simulink model "estimation_over_network"  (R2022b)
settings: Solver=VariableStepAuto  StartTime=0.0  StopTime=T  MaxStep=MaxStep  RelTol=RelTol
values from neighbouring files (symbols this model uses):
  J = 20    [initialization.m]
  T = 10    [initialization.m]
  X0 = [1;0.6;1]    [initialization.m]
libraries: HyEQ_Library x3
settings Model: Creator=tom  LastModifiedBy=tom

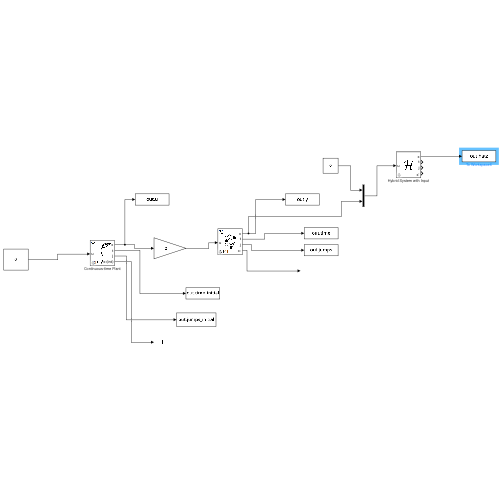
[thumbnail: Simulink's stored preview of the top-level diagram]
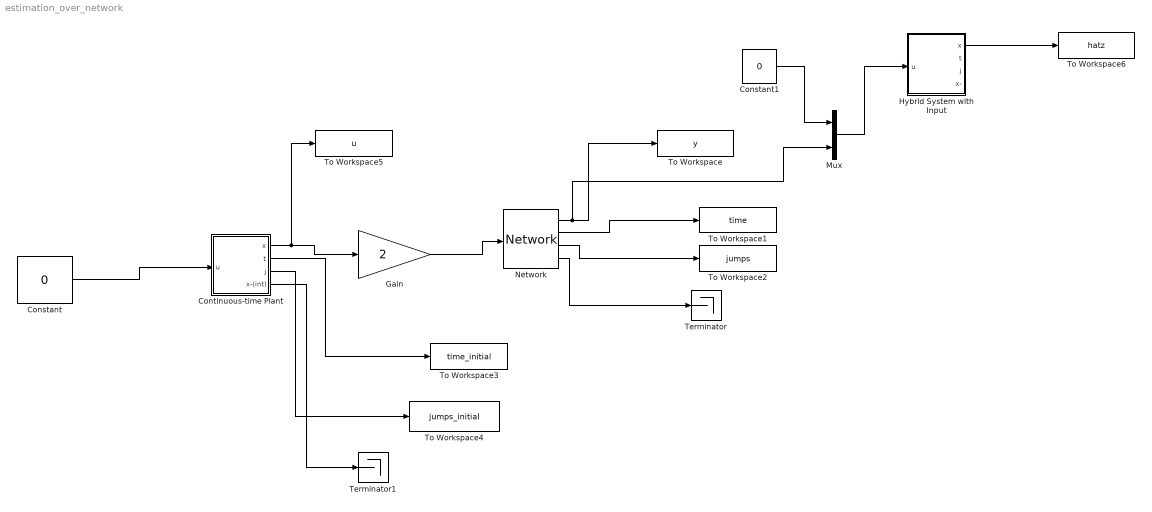
== system estimation_over_network ==
  Constant : Constant  Value=0
  Constant1 : Constant  Value=0
  Continuous-time Plant : Subsystem  LoadFcn=set_param(gcb,'LinkStatus','none')  mask(Continuous Process){z0=X0, input_dim=1, parameters=[], T=T}
      mask prompts: z0 "Initial State (column vector)"; input_dim "Input dimension (nonnegative integer)"; T "Flow Horizon (nonnegative real)"
      mask help:
      | To define the continuous process:
      | 1. Select the block,
      | 2. "Look inside" the block: Either open the context menu and select Mask > Look Under Mask, or click the arrow in the bottom-left corner of the block.
      | 3. Edit the "flow map f" block to define the continuous dynamics.
      | 4. Edit the "flow set C" block to define the region where the continuous process is allowed to flow.
      mask init:
      | state_dim = size(z0, 1);
      settings: CopyFcn=|
      | set_param(gcb,'LinkStatus','none'),
      | set_param(gcs, 'MaxStep', 'MaxStep', 'RelTol', 'RelTol','StopTime', 'T')
      mask Help: eval hybrid.internal.openHelp('Example_vehicle_on_path')
      mask TypeOptions T: Integrator System/T
      mask DialogControl Control2 Prompt: CPS Components Documentation
      mask DialogControl Control2 Callback: hybrid.internal.openHelp('CPS_Components')
      mask DialogControl ParameterGroupVar Prompt: Configuration
      mask Display:
      | image('Cplant.jpg')
      | port_label('output', 1, 'x')
      | port_label('output', 2, 't')
      | port_label('output', 3, 'j')
      | port_label('output', 4, 'x-(int)')
      | port_label('input', 1, 'u')
  Gain : Gain  Gain=2
  Hybrid System with Input : Subsystem  LoadFcn=set_param(gcb,'LinkStatus','none')  mask(Hybrid System with Inputs){x0=0, input_dim=6, parameters=[], T=T, J=J, rule=Jump}
      mask prompts: x0 "Initial Condition (column vector)"; input_dim "Input Dimension (positive integer)"; T "Flow Horizon (nonnegative real)"; J "Jump Horizon (nonnegative integer)"; rule "Flow/Jump Priorty Rule"
      mask help:
      | To modify (f, g, C, D) for this block, "Look inside" the block mask by either clicking the down arrow in the lower-left corner or selecting "Mask" > "Look Under Mask" from the context menu.
      |
      | For instructions how to use this block, see the
      mask init:
      | state_dim = numel(x0);
      settings: CopyFcn=|
      | set_param(gcb,'LinkStatus','none'),
      | set_param(gcs, 'MaxStep', 'MaxStep', 'RelTol', 'RelTol','StopTime', 'T')
      mask Help:
      | To modify (f, g, C, D) for this block, "Look inside" the block mask by either clicking the down arrow in the lower-left corner or selecting "Mask" > "Look Under Mask" from the context menu.
      | 
      | The value given in the 'parameters' field is passed as the last input argument for f, g, C, and D. Any MATLAB object can be used, but we recommend using a struct. For example, in the initialization script, a parameters struct can be defined as followed.
      |   parameters = struct();
      |   parameters.A = eye(2);
      |   parameters.B = [1; 0];
      | 
      | The output "x-" is the state output delayed by one integration step. Use this output to break algebraic loops.
      mask TypeOptions x0: Integrator System/x0
      mask TypeOptions T: Integrator System/T
      mask TypeOptions J: Integrator System/J
      mask TypeOptions rule: Jump | Flow | Random
      mask DialogControl Control2 Prompt: Introduction to the HyEQ Simulink-based Library
      mask DialogControl Control2 Callback: hybrid.internal.openHelp('Help_SimulinkLibrary')
      mask DialogControl Container3 Prompt: System Configuration
      mask DialogControl Container2 Prompt: Solver Options
      mask Display:
      | image('Hcal.jpg')
      | port_label('output', 1, 'x')
      | port_label('output', 2, 't')
      | port_label('output', 3, 'j')
      | port_label('output', 4, 'x^-','texmode', 'on')
      | port_label('input', 1, 'u')
  Mux : Mux  Inputs=2
  Network : HyEQ_Library/Cyber Physical Systems/Network  T_min=T_min  T_max=T_max  ms_0=y0  tau_0=tau_0  T=T  J=J
      settings: SourceProductName=Hybrid Equations Toolbox
  Terminator : Terminator
  Terminator1 : Terminator
  To Workspace : ToWorkspace  VariableName=y  SaveFormat=Timeseries  SampleTime=-1
  To Workspace1 : ToWorkspace  VariableName=time  SaveFormat=Timeseries  SampleTime=-1
  To Workspace2 : ToWorkspace  VariableName=jumps  SaveFormat=Timeseries  SampleTime=-1
  To Workspace3 : ToWorkspace  VariableName=time_initial  SaveFormat=Timeseries  SampleTime=-1
  To Workspace4 : ToWorkspace  VariableName=jumps_initial  SaveFormat=Timeseries  SampleTime=-1
  To Workspace5 : ToWorkspace  VariableName=u  SaveFormat=Timeseries  SampleTime=-1
  To Workspace6 : ToWorkspace  VariableName=hatz  SaveFormat=Timeseries  SampleTime=-1
  wires:
  Constant/1 -> Continuous-time Plant/1(u)
  Continuous-time Plant/1(x) -> To Workspace5/1, Gain/1
  Gain/1 -> Network/1
  Network/1 -> Mux/2, To Workspace/1
  Network/4 -> Terminator/1
  Network/3 -> To Workspace2/1
  Network/2 -> To Workspace1/1
  Continuous-time Plant/4(x-(int)) -> Terminator1/1
  Continuous-time Plant/2(t) -> To Workspace3/1
  Continuous-time Plant/3(j) -> To Workspace4/1
  Constant1/1 -> Mux/1
  Mux/1 -> Hybrid System with Input/1(u)
  Hybrid System with Input/1(x) -> To Workspace6/1

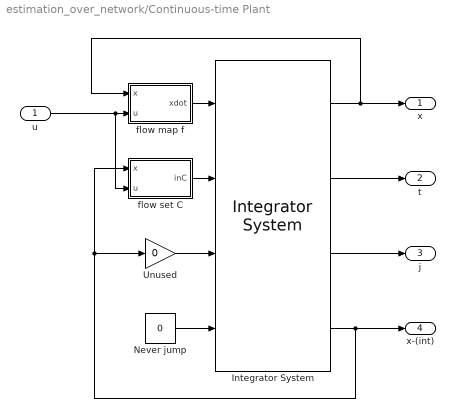
== system estimation_over_network/Continuous-time Plant ==
  u : Inport  PortDimensions=input_dim
  Integrator System : HyEQ_Library/Other/Integrator System  Priority=2  T=T  J=1  x0=z0  rule=1
      settings: SourceProductName=Hybrid Equations Toolbox
  Never jump : Constant  Value=0
  Unused : Gain  Gain=0
  flow map f : MATLAB Function  TreatAsAtomicUnit=on
  flow set C : MATLAB Function  TreatAsAtomicUnit=on
  x : Outport  PortDimensions=state_dim
  t : Outport  Port=2  PortDimensions=1
  j : Outport  Port=3  PortDimensions=1
  x-(int) : Outport  Port=4  PortDimensions=state_dim
  wires:
  Unused/1 -> Integrator System/3
  Never jump/1 -> Integrator System/4
  u/1 -> flow map f/2(u), flow set C/2(u)
  Integrator System/3 -> j/1
  Integrator System/2 -> t/1
  flow set C/1(inC) -> Integrator System/2
  Integrator System/1 -> x/1, flow map f/1(x)
  Integrator System/4 -> x-(int)/1, flow set C/1(x), Unused/1
  flow map f/1(xdot) -> Integrator System/1

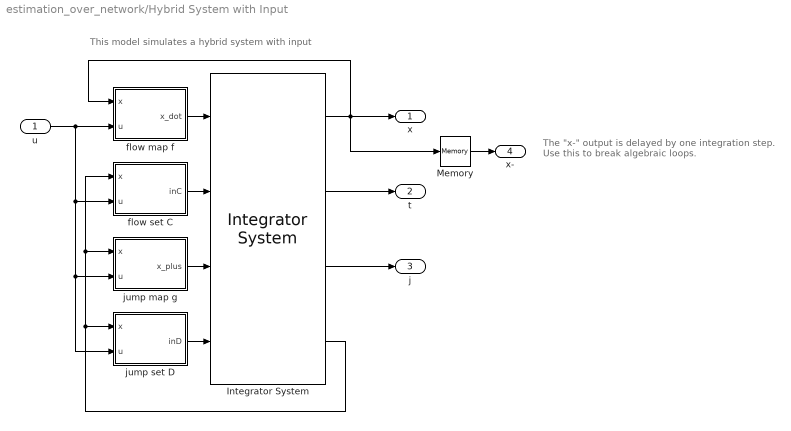
== system estimation_over_network/Hybrid System with Input ==
  note: This model simulates a hybrid system with input
  note: The "x-" output is delayed by one integration step. Use this to break algebraic loops.
  u : Inport  PortDimensions=input_dim
  Integrator System : HyEQ_Library/Other/Integrator System  Priority=2  T=T  J=J  x0=x0  rule=rule
      settings: SourceProductName=Hybrid Equations Toolbox
  Memory : Memory  InitialCondition=x0
  flow map f : MATLAB Function  TreatAsAtomicUnit=on
  flow set C : MATLAB Function  TreatAsAtomicUnit=on
  jump map g : MATLAB Function  TreatAsAtomicUnit=on
  jump set D : MATLAB Function  TreatAsAtomicUnit=on
  x : Outport  PortDimensions=state_dim
  t : Outport  Port=2  PortDimensions=1
  j : Outport  Port=3  PortDimensions=1
  x- : Outport  Port=4  PortDimensions=state_dim
  wires:
  Memory/1 -> x-/1
  jump map g/1(x_plus) -> Integrator System/3
  jump set D/1(inD) -> Integrator System/4
  u/1 -> jump set D/2(u), jump map g/2(u), flow set C/2(u), flow map f/2(u)
  Integrator System/3 -> j/1
  Integrator System/2 -> t/1
  flow set C/1(inC) -> Integrator System/2
  Integrator System/1 -> x/1, flow map f/1(x), Memory/1
  Integrator System/4 -> jump map g/1(x), flow set C/1(x), jump set D/1(x)
  flow map f/1(x_dot) -> Integrator System/1

== matlab function estimation_over_network/Hybrid System with Input/flow map f ==
  data: x input size=state_dim; u input size=input_dim; x_dot output size=state_dim
function x_dot = f(x, u)
   % Define flow map here.
   x_dot = -x + u(1);
end

== matlab function estimation_over_network/Hybrid System with Input/flow set C ==
  data: x input size=state_dim; u input size=input_dim; inC output size=1
function inC = C(x, u)
   % Define flow set indictor function here.
   inC = x >= u(1);
end

== matlab function estimation_over_network/Hybrid System with Input/jump map g ==
  data: x input size=state_dim; u input size=input_dim; x_plus output size=state_dim
function x_plus = g(x, u)
   % Jump map.
   x_plus = 10 + u(1);
end

== matlab function estimation_over_network/Hybrid System with Input/jump set D ==
  data: x input size=state_dim; u input size=input_dim; inD output size=1
function inD = D(x, u)
   % Define jump set indicator function here.
   inD = x <= u(1);
end

== matlab function estimation_over_network/Continuous-time Plant/flow map f ==
  data: x input size=state_dim; xdot output size=state_dim; u input size=input_dim
function xdot = f(x, u)
    % Define the flow map for the continuous process here.
    xdot_1 = -x(1) + u;
    xdot_2 = u + 1;
    xdot_3 = u - 2 + x(1);
    xdot = [xdot_1;xdot_2;xdot_3];
end

== matlab function estimation_over_network/Continuous-time Plant/flow set C ==
  data: x input size=state_dim; inC output size=1; u input size=input_dim
function inC = C(x, u)
    % Define the flow set indicator function for the continuous process here.
    inC = 1;
end
